simulink model "modele_avion_GPA745"  (R2016b)
settings: Solver=ode45  StartTime=0.0  StopTime=300  RelTol=1e-3  EnableMultiTasking=on
values from neighbouring files (symbols this model uses):
  A_lat = [-0.1094, 13.0137, -110.3137, 9.7483;   -0.0615, -1.8025, 0.9608, 0; 0.0024, -0.2635, -0.1127, 0;   0, 1, 0.1127, 0]    [labo5.m]
  A_lon = [ -0.0066, 0.1178, -12.5704, -9.7477;   -0.0910, -0.7560, 111.1563, -1.1037;   0.0055, -0.0477, -0.8536, 0; 0, 0, 1, 0]    [labo5.m]
  B_lat = [0, 1.2045; 2.3141, 0.3154; 0.2011, -0.3226; 0 0]    [labo5.m]
  B_lon = [0.4909; -6.0184; -2.5926; 0]    [labo5.m]
  freq = 0.117    [labo5.m]
  Ki = 30.0    (= 30)    [labo5.m]
  Kp = 0.3268    [labo5.m]
  Kq = -11.6667    [labo5.m]
  phase = 180    [labo5.m]
libraries: aerolibconvert2 x1, aerolibanim x1, aerolib6dofsys x1, aerolibtransform2 x1, aerolib6dof2 x1
settings Model: Creator=gghazi  LastModifiedBy=AP19030
settings DataIOCC: LimitDataPoints=on  SaveFormat=Array
settings OptimizationCC: LifeSpan=inf
settings DebuggingCC: UnderspecifiedInitializationDetection=Classic  MergeDetectMultiDrivingBlocksExec=none  SFUnexpectedBacktrackingDiag=warning  SFNoUnconditionalDefaultTransitionDiag=warning  SFExecutionAtInitializationDiag=none
settings HardwareCC: ProdBitPerPointer=32  ProdBitPerSizeT=32  ProdBitPerPtrDiffT=32  ProdLargestAtomicFloat=None  ProdIntDivRoundTo=Undefined  ProdEndianess=Unspecified  ProdWordSize=32  ProdHWDeviceType=32-bit Generic
settings ModelReferenceCC: PropagateSignalLabelsOutOfModel=off
settings GRTTargetCC: TargetLangStandard=C89/C90 (ANSI)  GeneratePreprocessorConditionals=Disable all
settings ConfigComp: CovMetricSettings=dw  CovHtmlReporting=on  CovSaveCumulativeToWorkspaceVar=on  CovSaveSingleToWorkspaceVar=on  CovExternalEMLEnable=off

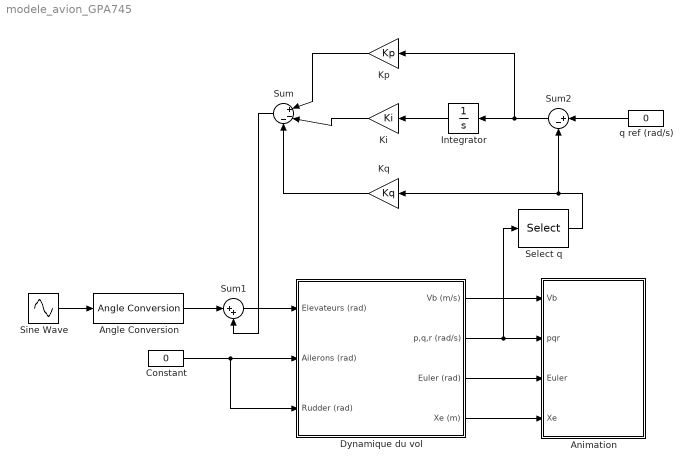
== system modele_avion_GPA745 ==
  Angle Conversion : aerolibconvert2/Angle Conversion  IU=deg  OU=rad
  Animation : Subsystem
  Constant : Constant  Value=0
  Dynamique du vol : Subsystem
  Integrator : Integrator
  Ki : Gain  Gain=Ki
  Kp : Gain  Gain=Kp
  Kq : Gain  Gain=Kq
  Select q : Selector  InputPortWidth=3  IndexOptions=Index vector (dialog)  Indices=[2]  OutputSizes=1
  Sine Wave : Sin  Frequency=freq  Phase=phase  SampleTime=300
  Sum : Sum  Inputs=|+--
  Sum1 : Sum  Inputs=|++
  Sum2 : Sum  Inputs=|+-
  q ref (rad/s) : Constant  Value=0
  wires:
  Dynamique du vol/3(Euler (rad)) -> Animation/3(Euler)
  Dynamique du vol/1(Vb (m/s)) -> Animation/1(Vb)
  Dynamique du vol/2(p,q,r (rad/s)) -> Select q/1, Animation/2(pqr)
  Dynamique du vol/4(Xe (m)) -> Animation/4(Xe)
  Constant/1 -> Dynamique du vol/3(Rudder (rad)), Dynamique du vol/2(Ailerons (rad))
  Sine Wave/1 -> Angle Conversion/1
  Select q/1 -> Sum2/2, Kq/1
  Kq/1 -> Sum/3
  Integrator/1 -> Ki/1
  Kp/1 -> Sum/1
  Ki/1 -> Sum/2
  Sum1/1 -> Dynamique du vol/1(Elevateurs (rad))
  Angle Conversion/1 -> Sum1/1
  Sum/1 -> Sum1/2
  Sum2/1 -> Kp/1, Integrator/1
  q ref (rad/s)/1 -> Sum2/1

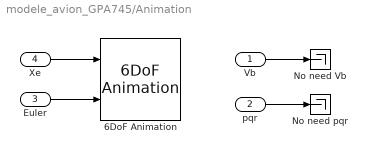
== system modele_avion_GPA745/Animation ==
  Vb : Inport
  pqr : Inport  Port=2
  Euler : Inport  Port=3
  Xe : Inport  Port=4
  6DoF Animation : aerolibanim/6DoF Animation  u1=[0 4000 -2000 2000 -5000 -3000]  u2=0.1  u3=50  u4=[0 0 0]  u5=Fly alongside  u6=[150 50 -30]/2  u7=50  u8=on
  No need Vb : Terminator
  No need pqr : Terminator
  wires:
  Euler/1 -> 6DoF Animation/2
  Vb/1 -> No need Vb/1
  pqr/1 -> No need pqr/1
  Xe/1 -> 6DoF Animation/1

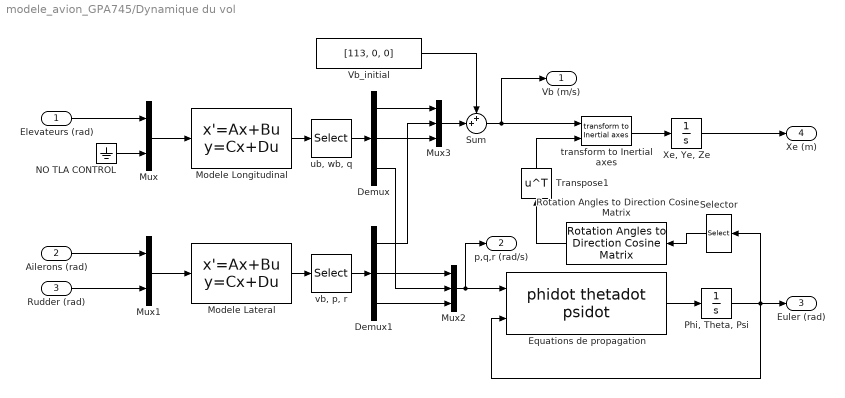
== system modele_avion_GPA745/Dynamique du vol ==
  Elevateurs (rad) : Inport
  Ailerons (rad) : Inport  Port=2
  Rudder (rad) : Inport  Port=3
  Demux : Demux  Outputs=3
  Demux1 : Demux  Outputs=3
  Equations de propagation : aerolib6dofsys/DCM & Euler Angles (Euler)/phidot thetadot psidot
  Modele Lateral : StateSpace  A=A_lat  B=B_lat  C=eye(4)  D=zeros(4,2)  X0=[0, 0, 0, 0]
  Modele Longitudinal : StateSpace  A=A_lon  B=[B_lon(:,1), zeros(4,1)]  C=eye(4)  D=zeros(4,2)  X0=[0, 0, 0, 0]
  Mux : Mux  Inputs=2
  Mux1 : Mux  Inputs=2
  Mux2 : Mux  Inputs=3
  Mux3 : Mux  Inputs=3
  NO TLA CONTROL : Ground
  "Phi, Theta, Psi" : Integrator  InitialCondition=[0,0,0]
  Rotation Angles to Direction Cosine Matrix : aerolibtransform2/Rotation Angles to Direction Cosine Matrix  rotationOrder=ZYX
  Selector : Selector  InputPortWidth=3  IndexOptions=Index vector (dialog)  Indices=[3 2 1]  OutputSizes=1
  Sum : Sum  Inputs=++|
  Transpose1 : Math  Operator=transpose  SaturateOnIntegerOverflow=on
  Vb_initial : Constant  Value=[113, 0, 0]
  "Xe, Ye, Ze" : Integrator  InitialCondition=[0,0 -4572]
  "transform to Inertial axes " : aerolib6dof2/6DOF (Euler Angles)/transform to Inertial axes   SystemSampleTime=-1
  "ub, wb, q" : Selector  InputPortWidth=4  IndexOptions=Index vector (dialog)  Indices=[1 2 3]  OutputSizes=1
  "vb, p, r" : Selector  InputPortWidth=4  IndexOptions=Index vector (dialog)  Indices=[1 2 3]  OutputSizes=1
  Vb (m/s) : Outport
  p,q,r (rad/s) : Outport  Port=2
  Euler (rad) : Outport  Port=3
  Xe (m) : Outport  Port=4
  wires:
  Mux/1 -> Modele Longitudinal/1
  Elevateurs (rad)/1 -> Mux/1
  Mux1/1 -> Modele Lateral/1
  Ailerons (rad)/1 -> Mux1/1
  Rudder (rad)/1 -> Mux1/2
  NO TLA CONTROL/1 -> Mux/2
  Modele Longitudinal/1 -> "ub, wb, q"/1
  Modele Lateral/1 -> "vb, p, r"/1
  "Phi, Theta, Psi"/1 -> Equations de propagation/2, Euler (rad)/1, Selector/1
  Equations de propagation/1 -> "Phi, Theta, Psi"/1
  "ub, wb, q"/1 -> Demux/1
  "vb, p, r"/1 -> Demux1/1
  Demux/1 -> Mux3/1
  Demux/2 -> Mux3/3
  Demux1/1 -> Mux3/2
  Demux1/3 -> Mux2/3
  Demux1/2 -> Mux2/1
  Demux/3 -> Mux2/2
  Mux2/1 -> Equations de propagation/1, p,q,r (rad/s)/1
  Transpose1/1 -> "transform to Inertial axes "/2
  Rotation Angles to Direction Cosine Matrix/1 -> Transpose1/1
  Selector/1 -> Rotation Angles to Direction Cosine Matrix/1
  "transform to Inertial axes "/1 -> "Xe, Ye, Ze"/1
  "Xe, Ye, Ze"/1 -> Xe (m)/1
  Mux3/1 -> Sum/2
  Vb_initial/1 -> Sum/1
  Sum/1 -> "transform to Inertial axes "/1, Vb (m/s)/1
